simulink model "example_dynamics"  (R2016a)
settings: Solver=VariableStepAuto  StartTime=0.0  StopTime=60  RelTol=1e-3
libraries: simulink x1
settings Model: Creator=mgreiff  LastModifiedBy=mgreiff

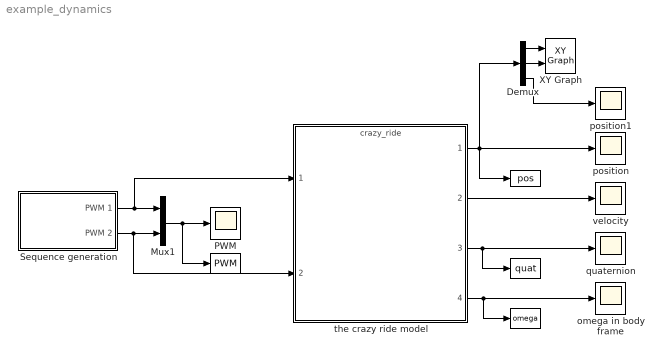
== system example_dynamics ==
  "  " : ToWorkspace  VariableName=quat  SaveFormat=Timeseries  SampleTime=-1
  "   " : ToWorkspace  VariableName=PWM  SaveFormat=Timeseries  SampleTime=-1
  "    " : ToWorkspace  VariableName=omega  SaveFormat=Timeseries  SampleTime=-1
  "     " : ToWorkspace  VariableName=pos  SaveFormat=Timeseries  SampleTime=-1
  Demux : Demux  Outputs=[1,1,1]
  Mux1 : Mux  Inputs=2
  PWM : Scope
  Sequence generation : Subsystem
  XY Graph : simulink/Sinks/XY Graph  xmin=-1  xmax=1  ymin=-1  ymax=1  st=-1
  omega in body frame : Scope
  position : Scope
  position1 : Scope
  quaternion : Scope
  the crazy ride model : ModelReference  ModelNameDialog=crazy_ride.slx  SimulationMode=Normal  ModelReferenceVersion=1.12
  velocity : Scope
  wires:
  the crazy ride model/1 -> position/1, "     "/1, Demux/1
  the crazy ride model/4 -> omega in body frame/1, "    "/1
  the crazy ride model/3 -> "  "/1, quaternion/1
  the crazy ride model/2 -> velocity/1
  Demux/1 -> XY Graph/1
  Demux/2 -> XY Graph/2
  Demux/3 -> position1/1
  Sequence generation/1(PWM 1) -> Mux1/1, the crazy ride model/1
  Sequence generation/2(PWM 2) -> Mux1/2, the crazy ride model/2
  Mux1/1 -> "   "/1, PWM/1

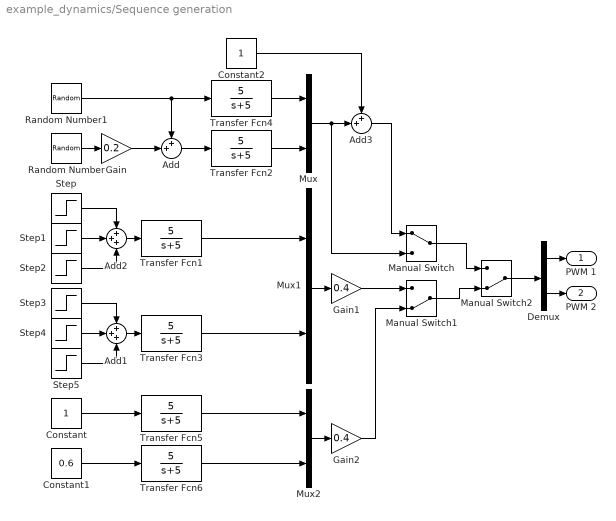
== system example_dynamics/Sequence generation ==
  Add : Sum  Inputs=++|
  Add1 : Sum  Inputs=+++
  Add2 : Sum  Inputs=+++
  Add3 : Sum  Inputs=++|
  Constant : Constant
  Constant1 : Constant  Value=0.6
  Constant2 : Constant
  Demux : Demux  Outputs=2
  Gain : Gain  Gain=0.2
  Gain1 : Gain  Gain=0.4
  Gain2 : Gain  Gain=0.4
  Manual Switch : ManualSwitch
  Manual Switch1 : ManualSwitch  CurrentSetting=0
  Manual Switch2 : ManualSwitch  CurrentSetting=0
  Mux : Mux  Inputs=2
  Mux1 : Mux  Inputs=2
  Mux2 : Mux  Inputs=2
  Random Number : RandomNumber  Seed=1  SampleTime=1
  Random Number1 : RandomNumber  SampleTime=1
  Step : Step  SampleTime=0
  Step1 : Step  Time=3  After=-2  SampleTime=0
  Step2 : Step  Time=5  SampleTime=0
  Step3 : Step  Time=7  SampleTime=0
  Step4 : Step  Time=9  After=-2  SampleTime=0
  Step5 : Step  Time=11  SampleTime=0
  Transfer Fcn{1..6} (6 alike) : TransferFcn  Numerator=[5]  Denominator=[1 5]
  PWM 1 : Outport
  PWM 2 : Outport  Port=2
  wires:
  Random Number1/1 -> Transfer Fcn4/1, Add/1
  Gain/1 -> Add/2
  Random Number/1 -> Gain/1
  Add/1 -> Transfer Fcn2/1
  Step/1 -> Add2/1
  Step1/1 -> Add2/2
  Step2/1 -> Add2/3
  Step4/1 -> Add1/2
  Step3/1 -> Add1/1
  Step5/1 -> Add1/3
  Mux1/1 -> Gain1/1
  Demux/2 -> PWM 2/1
  Demux/1 -> PWM 1/1
  Manual Switch2/1 -> Demux/1
  Add2/1 -> Transfer Fcn1/1
  Transfer Fcn1/1 -> Mux1/1
  Add1/1 -> Transfer Fcn3/1
  Transfer Fcn3/1 -> Mux1/2
  Transfer Fcn4/1 -> Mux/1
  Transfer Fcn2/1 -> Mux/2
  Constant/1 -> Transfer Fcn5/1
  Constant1/1 -> Transfer Fcn6/1
  Transfer Fcn5/1 -> Mux2/1
  Transfer Fcn6/1 -> Mux2/2
  Mux2/1 -> Gain2/1
  Gain2/1 -> Manual Switch1/2
  Gain1/1 -> Manual Switch1/1
  Manual Switch1/1 -> Manual Switch2/2
  Mux/1 -> Add3/2, Manual Switch/2
  Manual Switch/1 -> Manual Switch2/1
  Add3/1 -> Manual Switch/1
  Constant2/1 -> Add3/1
